simulink model "mdlRef2"  (R2023b)
settings: Solver=VariableStepAuto  StartTime=0.0  StopTime=10.0  RelTol=1e-3
settings Model: Creator=neham  LastModifiedBy=neham

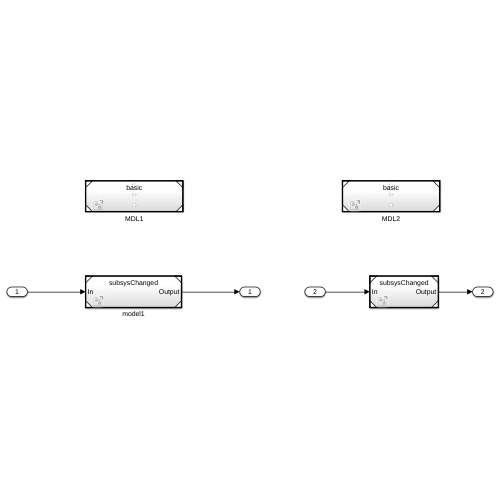
[thumbnail: Simulink's stored preview of the top-level diagram]
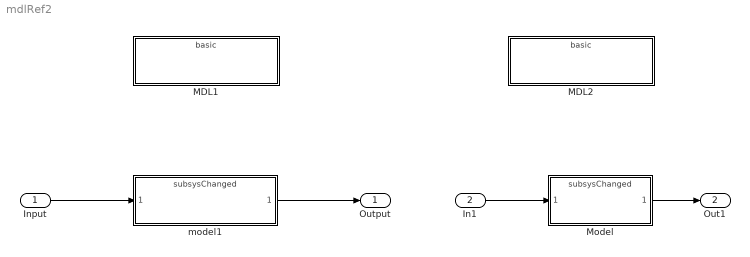
== system mdlRef2 ==
  Input : Inport
  In1 : Inport  Port=2
  MDL1 : ModelReference  ModelNameDialog=basic.slx  SimulationMode=Normal  ModelReferenceVersion=1.4
  MDL2 : ModelReference  ModelNameDialog=basic.slx  SimulationMode=Normal  ModelReferenceVersion=1.4
  Model : ModelReference  ModelNameDialog=subsysChanged.slx  SimulationMode=Normal  ModelReferenceVersion=1.1
  model1 : ModelReference  ModelNameDialog=subsysChanged.slx  SimulationMode=Normal  ModelReferenceVersion=1.1
  Output : Outport
  Out1 : Outport  Port=2
  wires:
  Input/1 -> model1/1
  model1/1 -> Output/1
  In1/1 -> Model/1
  Model/1 -> Out1/1
